simulink model "MBDques6"  (R2020a)
settings: Solver=VariableStepAuto  StartTime=0.0  StopTime=10.0  RelTol=1e-3
settings Model: Creator=DELL  LastModifiedBy=DELL

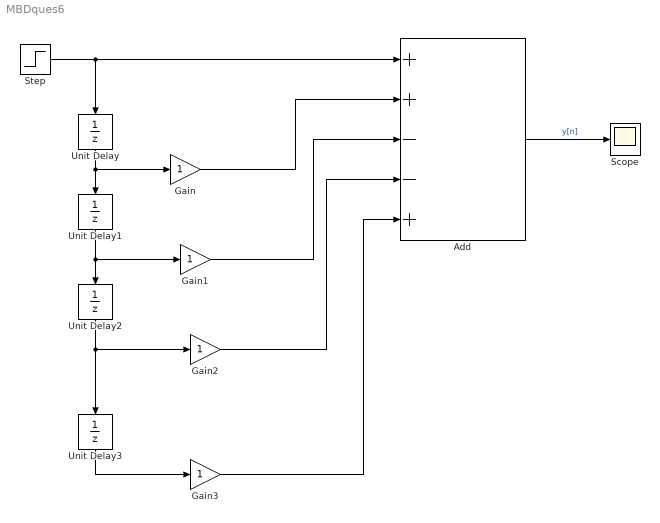
== system MBDques6 ==
  Add : Sum  Inputs=++--+
  Gain{,1..3} (4 alike) : Gain
  Scope : Scope
  Step : Step  SampleTime=0
  Unit Delay{,1..3} (4 alike) : UnitDelay  SampleTime=-1  HasFrameUpgradeWarning=on
  wires:
  Step/1 -> Unit Delay/1, Add/1
  Unit Delay/1 -> Unit Delay1/1, Gain/1
  Gain/1 -> Add/2
  Unit Delay1/1 -> Unit Delay2/1, Gain1/1
  Gain1/1 -> Add/3
  Unit Delay2/1 -> Unit Delay3/1, Gain2/1
  Gain2/1 -> Add/4
  Unit Delay3/1 -> Gain3/1
  Gain3/1 -> Add/5
  Add/1 -> Scope/1  "y[n]"
